simulink model "Vehicle_Dynamics"  (R2025b)
settings: Solver=VariableStepAuto  StartTime=0.0  StopTime=10.0  RelTol=1e-3
undefined symbols (not defined in the file or in its folder): distMode
settings Model: Creator=andrew  LastModifiedBy=andrew

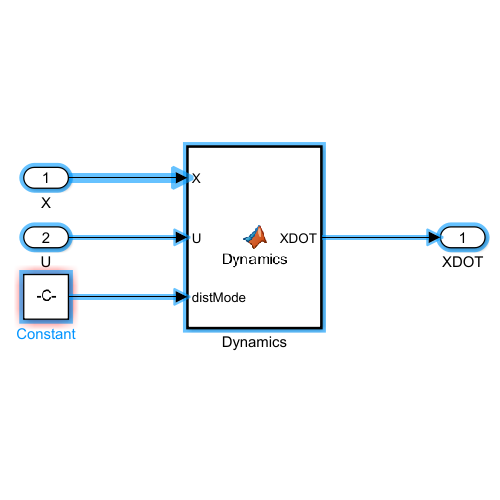
[thumbnail: Simulink's stored preview of the top-level diagram]
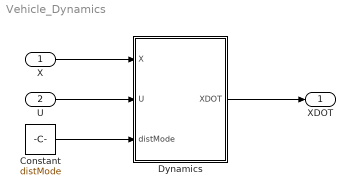
== system Vehicle_Dynamics ==
  X : Inport
  U : Inport  Port=2
  Constant : Constant  Value=distMode
  Dynamics : MATLAB Function  TreatAsAtomicUnit=on
  XDOT : Outport
  wires:
  U/1 -> Dynamics/2(U)
  Constant/1 -> Dynamics/3(distMode)
  Dynamics/1(XDOT) -> XDOT/1
  X/1 -> Dynamics/1(X)

== matlab function Vehicle_Dynamics/Dynamics ==
  data: X input; XDOT output; U input; distMode input
function XDOT = Dynamics(X, U, distMode)
if distMode == 1
    XDOT = disturbedDynamics(X, U);
else
    XDOT = nominalDynamics(X, U);
end
